simulink model "PWM_STM32_g431xx_Boost_Converter_Controller"  (R2025b)
settings: Solver=FixedStepAuto  StartTime=0.0  StopTime=inf  FixedStep=Ts  RelTol=1e-3  EnableMultiTasking=on
InitFcn:
  | Startup_Parameters
values from neighbouring files (symbols this model uses):
  ARR = (Fclk/Dpwm) - 1    (= 339)    [Startup_Parameters.m]
  K1 = Kp + alpha*Ts*Ki    (= 0.0202)    [Startup_Parameters.m]
  K2 = Ts*Ki    (= 0.0004)    [Startup_Parameters.m]
  Ts = 1e-5    (= 1e-05)    [Startup_Parameters.m]    (also in Transfer_Functions_Boost_STM32.m = 2e-06)
libraries: stm32f4xxblockslib x2
settings Model: STM32="{\"DigitalPortWrite\":[{\"ID\":\"Blinky:1\"},{\"ID\":\"Blinky_Chidote:1\"},{\"ID\":\"PWM_STM32_g431xx:1\"},{\"ID\":\"PWM_STM32_g431xx_Boost_Converter:1\"},{\"ID\":\"PWM_STM32_g431xx_Boost_Converter:13\"}],\"PWMOutput\":[{\"ID\":\"Blinky_Chidote:3\"},{\"ID\":\"PWM_STM32_g431xx:3\"},{\"ID\":\"PWM_STM32_g431xx_Boost_Converter:3\"},{\"ID\":\"PWM_STM32_g431xx_Boost_Converter_Controller:3\"}],\"AnalogInput\":[{\"ID\":\"PWM_STM32_g431xx_Boost_Converter:35\"},{\"ID\":\"PWM_STM32_g431xx_Boost_Converter_Controller:35\"}]}"  Creator=Erick Negrete  LastModifiedBy=Erick Negrete
settings OptimizationCC: EnhancedBackFolding=on  PassReuseOutputArgsAs=Individual arguments  ZeroExternalMemoryAtStartup=off  ZeroInternalMemoryAtStartup=off  MaxStackSize=512  OptimizeBlockOrder=speed  DifferentSizesBufferReuse=on  OptimizationCustomize=off  EfficientTunableParamExpr=on
settings DebuggingCC: ParameterTunabilityLossMsg=error
settings HardwareCC: ProdBitPerPointer=32.0  ProdBitPerSizeT=32.0  ProdBitPerPtrDiffT=32.0  ProdLargestAtomicInteger=Long  ProdLargestAtomicFloat=Double  ProdWordSize=32.0  ProdLongLongMode=on  ProdHWDeviceType=ARM Compatible->ARM Cortex-M
settings SFSimCC: MATLABDynamicMemAlloc=off
settings RTWCC: SystemTargetFile=ert.tlc  HardwareBoard=STM32G4xx Based  TemplateMakefile=ert_default_tmf  Toolchain=GNU Tools for ARM Embedded Processors  IncludeHyperlinkInReport=on  Description=Embedded Coder
settings CodeAppCC: ForceParamTrailComments=on  IgnoreCustomStorageClasses=off  OperatorAnnotations=on  SimulinkDataObjDesc=on  SFDataObjDesc=on  InsertBlockDesc=on
settings ERTTargetCC: ExtModeTransport=3.0  ExtModeStaticAlloc=on  ExtModeStaticAllocSize=10000.0  ExtModeMexFile=ext_xcp  ExtModeIntrfLevel=Level2 - Open  InlinedParameterPlacement=Hierarchical  TargetLangStandard=C99 (ISO)  CodeReplacementLibrary=ARM Cortex-M

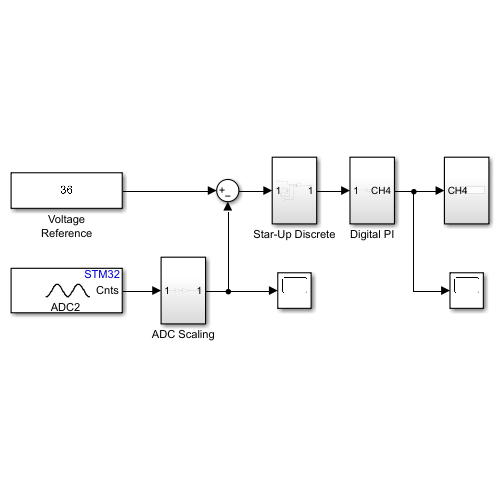
[thumbnail: Simulink's stored preview of the top-level diagram]
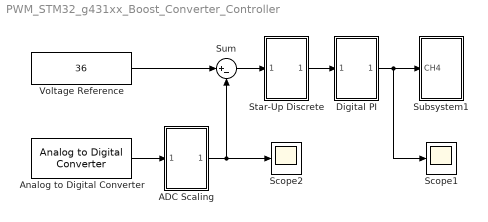
== system PWM_STM32_g431xx_Boost_Converter_Controller ==
  ADC Scaling : Subsystem
  Analog to Digital Converter : stm32f4xxblockslib/Analog to Digital Converter  ADCModule=ADC2  ConversionGroup=Regular  TriggerMode=Trigger and read  NumberOfConversions=1  EnableBufferConv=off  BufferLength=1  OutputStatus=off  SampleTime=Ts  EnableSimPort=off  hoistedMaskSrc=ECSoC/ECSimCodegen/Analog to Digital Converter
  Digital PI : Subsystem
  Scope1 : Scope
      settings: ActiveDisplayYMinimum=-1  ActiveDisplayYMaximum=1
  Scope2 : Scope
      settings: ActiveDisplayYMinimum=23.550602793693542  ActiveDisplayYMaximum=23.620107769966125
  Star-Up Discrete : Subsystem
  Subsystem1 : Subsystem
  Sum : Sum  Inputs=|+-
  Voltage Reference : Constant  Value=36
  wires:
  Voltage Reference/1 -> Sum/1
  Sum/1 -> Star-Up Discrete/1(In1)
  Star-Up Discrete/1(Out1) -> Digital PI/1(In1)
  ADC Scaling/1(Out1) -> Scope2/1, Sum/2
  Analog to Digital Converter/1 -> ADC Scaling/1(In1)
  Digital PI/1(CH4) -> Scope1/1, Subsystem1/1(CH4)

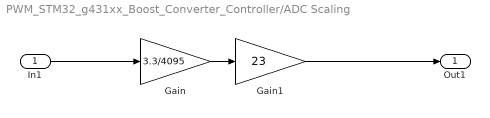
== system PWM_STM32_g431xx_Boost_Converter_Controller/ADC Scaling ==
  In1 : Inport
  Gain : Gain  Gain=3.3/4095
  Gain1 : Gain  Gain=23
  Out1 : Outport
  wires:
  Gain/1 -> Gain1/1
  In1/1 -> Gain/1
  Gain1/1 -> Out1/1

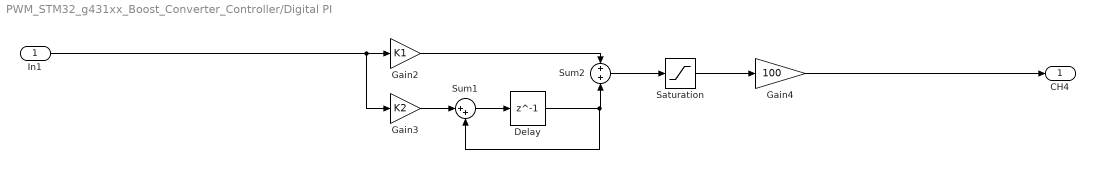
== system PWM_STM32_g431xx_Boost_Converter_Controller/Digital PI ==
  In1 : Inport
  Delay : Delay  DelayLength=1  SampleTime=Ts
  Gain2 : Gain  Gain=K1
  Gain3 : Gain  Gain=K2
  Gain4 : Gain  Gain=100
  Saturation : Saturate  UpperLimit=0.8  LowerLimit=0
  Sum1 : Sum  Inputs=|++
  Sum2 : Sum  Inputs=+|+
  CH4 : Outport
  wires:
  Delay/1 -> Sum1/2, Sum2/2
  Sum1/1 -> Delay/1
  Gain2/1 -> Sum2/1
  Gain3/1 -> Sum1/1
  Sum2/1 -> Saturation/1
  Gain4/1 -> CH4/1
  Saturation/1 -> Gain4/1
  In1/1 -> Gain3/1, Gain2/1

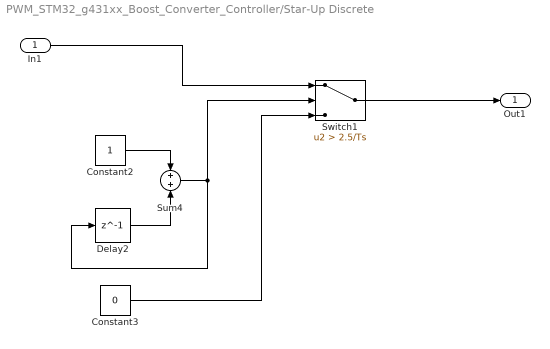
== system PWM_STM32_g431xx_Boost_Converter_Controller/Star-Up Discrete ==
  In1 : Inport
  Constant2 : Constant
  Constant3 : Constant  Value=0
  Delay2 : Delay  DelayLength=1  SampleTime=Ts
  Sum4 : Sum
  Switch1 : Switch  Criteria=u2 > Threshold  Threshold=2.5/Ts  SaturateOnIntegerOverflow=off  InputSameDT=off
  Out1 : Outport
  wires:
  Delay2/1 -> Sum4/2
  Constant3/1 -> Switch1/3
  Constant2/1 -> Sum4/1
  Sum4/1 -> Switch1/2, Delay2/1
  Switch1/1 -> Out1/1
  In1/1 -> Switch1/1

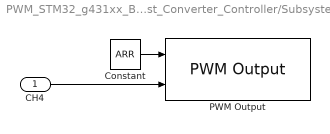
== system PWM_STM32_g431xx_Boost_Converter_Controller/Subsystem1 ==
  CH4 : Inport
  Constant : Constant  Value=ARR
  PWM Output : stm32f4xxblockslib/PWM Output  ProcessorFamily=STM32G4  TimerModule=TIM2  DutycycleUnits=Percentage  EnableChannel1=off  EnableCaptureCompare1Input=off  EnableCaptureCompare1ComplementaryInput=off  EnableOutputCompare1ModeInput=off  EnableChannel2=off  EnableCaptureCompare2Input=off  EnableCaptureCompare2ComplementaryInput=off  EnableOutputCompare2ModeInput=off  EnableChannel3=off  EnableCaptureCompare3Input=off  EnableCaptureCompare3ComplementaryInput=off  EnableOutputCompare3ModeInput=off  EnableChannel4=on  EnableCaptureCompare4Input=off  EnableCaptureCompare4ComplementaryInput=off  EnableOutputCompare4ModeInput=off  EnableChannel5=off  EnableCaptureCompare5Input=off  EnableOutputCompare5ModeInput=off  EnableChannel6=off  EnableCaptureCompare6Input=off  EnableOutputCompare6ModeInput=off  EnableCounterInput=off  EnableMainOutputInput=off  EnableFrequencyInput=on  SetRCAfterCE=off  OutputDirection=off  OutputMainOutputEnableStatus=off  SampleTime=0.1  EnableSimPort=off  EnableUpdateEvent=off  EnableCaptureCompare1Event=off  EnableCaptureCompare2Event=off  EnableCaptureCompare3Event=off  EnableCaptureCompare4Event=off  EnableTriggerEvent=off  EnableBreakEvent=off  EnableBreakEvent2=off  hoistedMaskSrc=ECSoC/ECSimCodegen/PWM Output
      settings: LibrarySourceBlock=stm32g4xxblockslib/PWM Output
  wires:
  Constant/1 -> PWM Output/1
  CH4/1 -> PWM Output/2
